simulink model "Bouncingball"  (R2024b)
settings: Solver=VariableStepAuto  StartTime=0.0  StopTime=25  RelTol=1e-3
settings Model: Creator=rares  LastModifiedBy=rares

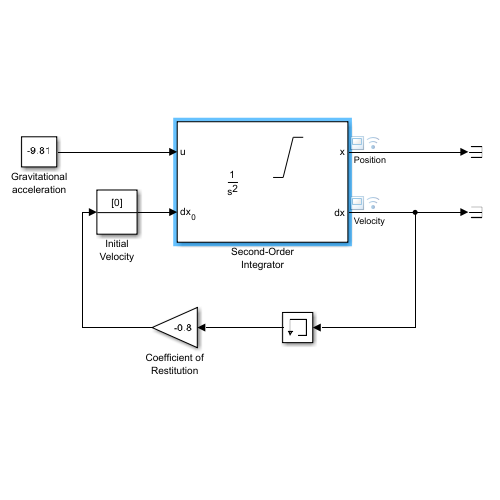
[thumbnail: Simulink's stored preview of the top-level diagram]
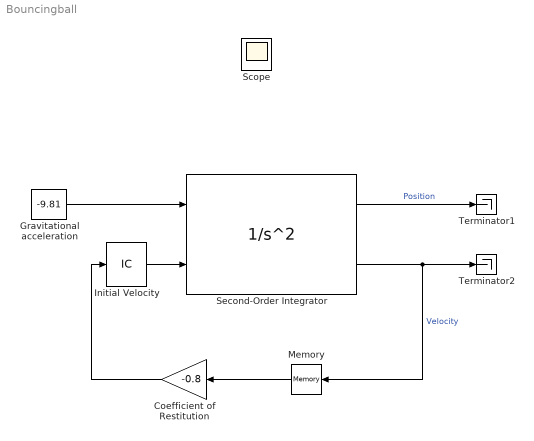
== system Bouncingball ==
  Coefficient of Restitution : Gain  Gain=-0.8
  Gravitational acceleration : Constant  Value=-9.81
  Initial Velocity : InitialCondition  Value=0
  Memory : Memory
  Second-Order Integrator : SecondOrderIntegrator  ICX=25.0  LimitX=on  LowerLimitX=0.0  StateNameX='Position'  ICSourceDXDT=external  StateNameDXDT='Velocity'  ReinitDXDTwhenXreachesSaturation=on
  Terminator1 : Terminator
  Terminator2 : Terminator
  Scope : Scope
  wires:
  Gravitational acceleration/1 -> Second-Order Integrator/1
  Second-Order Integrator/1 -> Terminator1/1  "Position"
  Initial Velocity/1 -> Second-Order Integrator/2
  Coefficient of Restitution/1 -> Initial Velocity/1
  Memory/1 -> Coefficient of Restitution/1
  Second-Order Integrator/2 -> Terminator2/1, Memory/1  "Velocity"
